simulink model "simulink_case"  (R2024b)
settings: Solver=ode1  StartTime=0.0  StopTime=T  FixedStep=dt  RelTol=1e-3
undefined symbols (not defined in the file or in its folder): DiscIntNeverNeededParam
settings Model: Creator=aalessan  LastModifiedBy=aalessan

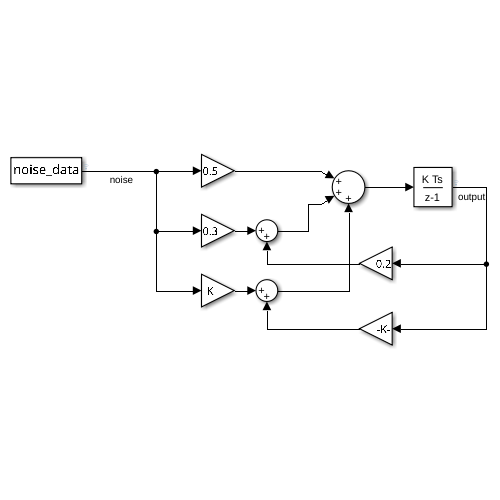
[thumbnail: Simulink's stored preview of the top-level diagram]
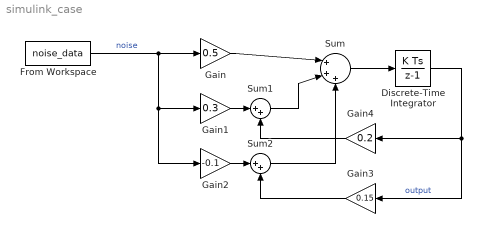
== system simulink_case ==
  Discrete-Time Integrator : DiscreteIntegrator  SampleTime=-1  ICPrevOutput=DiscIntNeverNeededParam  ICPrevScaledInput=DiscIntNeverNeededParam
  From Workspace : FromWorkspace  VariableName=noise_data  Interpolate=off  OutputAfterFinalValue=Setting to zero
  Gain : Gain  Gain=0.5
  Gain1 : Gain  Gain=0.3
  Gain2 : Gain  Gain=-0.1
  Gain3 : Gain  Gain=0.15
  Gain4 : Gain  Gain=0.2
  Sum : Sum  Inputs=|+++
  Sum1 : Sum  Inputs=|++
  Sum2 : Sum  Inputs=|++
  wires:
  From Workspace/1 -> Gain2/1, Gain1/1, Gain/1  "noise"
  Gain/1 -> Sum/1
  Gain1/1 -> Sum1/1
  Sum1/1 -> Sum/2
  Gain2/1 -> Sum2/1
  Sum2/1 -> Sum/3
  Sum/1 -> Discrete-Time Integrator/1
  Discrete-Time Integrator/1 -> Gain4/1, Gain3/1  "output"
  Gain3/1 -> Sum2/2
  Gain4/1 -> Sum1/2
